simulink model "MotorEC"  (R2013b)
settings: Solver=ode45  StartTime=0.0  StopTime=10.0  RelTol=1e-3
settings Model: Creator=Eduardo  LastModifiedBy=Eduardo

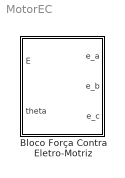
== system MotorEC ==
  "Bloco Força Contra Eletro-Motriz " : Subsystem

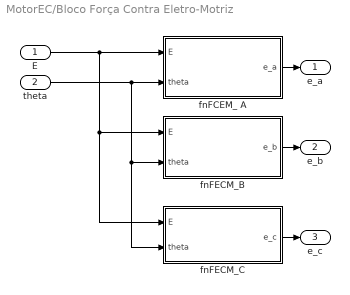
== system MotorEC/Bloco Força Contra Eletro-Motriz  ==
  E : Inport
  theta : Inport  Port=2
  fnFCEM_ A : MATLAB Function  TreatAsAtomicUnit=on
  "fnFECM_B " : MATLAB Function  TreatAsAtomicUnit=on
  "fnFECM_C " : MATLAB Function  TreatAsAtomicUnit=on
  e_a : Outport
  e_b : Outport  Port=2
  e_c : Outport  Port=3
  wires:
  "fnFECM_C "/1(e_c) -> e_c/1
  "fnFECM_B "/1(e_b) -> e_b/1
  theta/1 -> "fnFECM_C "/2(theta), "fnFECM_B "/2(theta), fnFCEM_ A/2(theta)
  E/1 -> "fnFECM_C "/1(E), "fnFECM_B "/1(E), fnFCEM_ A/1(E)
  fnFCEM_ A/1(e_a) -> e_a/1

== matlab function MotorEC/Bloco Força Contra Eletro-Motriz /fnFECM_B  ==
  data: E input; e_b output; theta input
function e_b = fnFCEM_B (E, theta)

% Cálculo da força eletromotriz no ramo A.
% ----------------------------------------

if (0 < theta && theta <= pi/2)
   e_b = -E;
end

if (pi/2 < theta && theta <= (5*pi)/6)
   e_b = (6*E/pi)*theta - 4*E;
end

if ((5*pi)/6 < theta && theta <= (9*pi)/6)
   e_b = E;
end

if ((9*pi)/6 < theta && theta <= (11*pi)/6)
   e_b = -(6*E/pi)*theta + 10*E;
end

if ((11*pi)/6 < theta && theta <= 2*pi)
   e_b = -E;
end

end

== matlab function MotorEC/Bloco Força Contra Eletro-Motriz /fnFCEM_ A ==
  data: E input; e_a output; theta input
function e_a = fnFCEM_A (E, theta)

% Cálculo da força eletromotriz no ramo A.
% ----------------------------------------

if (0 < theta && theta <= pi/6)
   e_a = (6*E/pi)*theta;
end

if (pi/6 < theta && theta <= (5*pi)/6)
   e_a = E;
end

if ((5*pi)/6 < theta && theta <= (7*pi)/6)
   e_a = -(6*E/pi)*theta + 6*E;
end

if ((7*pi)/6 < theta && theta <= (11*pi)/6)
   e_a = -E;
end

if ((11*pi)/6 < theta && theta <= 2*pi)
   e_a = (6*E/pi)*theta - 12*E;
end

end

== matlab function MotorEC/Bloco Força Contra Eletro-Motriz /fnFECM_C  ==
  data: E input; e_c output; theta input
function e_c = fnFCEM_C (E, theta)

% Cálculo da força eletromotriz no ramo A.
% ----------------------------------------

if (0 < theta && theta <= pi/6)
   e_c = E;
end

if (pi/6 < theta && theta <= pi/2)
   e_c = -(6*E/pi)*theta + 2*E;
end

if (pi/2 < theta && theta <= (7*pi)/6)
   e_c = -E;
end

if ((7*pi)/6 < theta && theta <= (9*pi)/6)
   e_c = (6*E/pi)*theta - 8*E;
end

if ((9*pi)/6 < theta && theta <= 2*pi)
   e_c = E;
end

end
